simulink library "mdderslib_conversions"  (Simulink 7.8)
settings: Solver=ode45  StartTime=0.0  StopTime=10.0  RelTol=1e-3
settings Model: Creator=Tomas  LastModifiedBy=bures

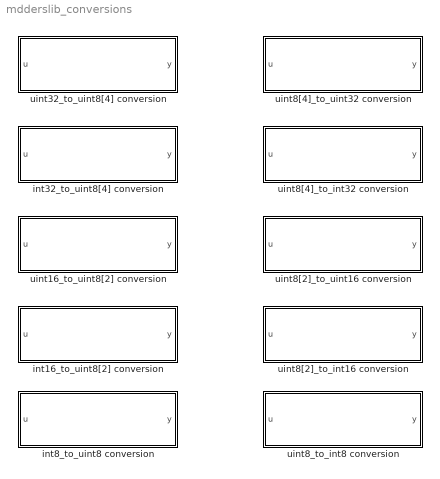
== system mdderslib_conversions ==
  int16_to_uint8[2] conversion : MATLAB Function  TreatAsAtomicUnit=on
  int32_to_uint8[4] conversion : MATLAB Function  TreatAsAtomicUnit=on
  int8_to_uint8 conversion : MATLAB Function  TreatAsAtomicUnit=on
  uint16_to_uint8[2] conversion : MATLAB Function  TreatAsAtomicUnit=on
  uint32_to_uint8[4] conversion : MATLAB Function  TreatAsAtomicUnit=on
  uint8[2]_to_int16 conversion : MATLAB Function  TreatAsAtomicUnit=on
  uint8[2]_to_uint16 conversion : MATLAB Function  TreatAsAtomicUnit=on
  uint8[4]_to_int32 conversion : MATLAB Function  TreatAsAtomicUnit=on
  uint8[4]_to_uint32 conversion : MATLAB Function  TreatAsAtomicUnit=on
  uint8_to_int8 conversion : MATLAB Function  TreatAsAtomicUnit=on

== matlab function uint32_to_uint8[4] conversion ==
  data: u input uint32 size=[1 1]; y output uint8 size=[1 4]
function y = uint32_to_uint8(u)
%#codegen

y = typecast(uint32(u), 'uint8');

== matlab function int32_to_uint8[4] conversion ==
  data: u input int32 size=[1 1]; y output uint8 size=[1 4]
function y = int32_to_uint8(u)
%#codegen

y = typecast(int32(u), 'uint8');

== matlab function int16_to_uint8[2] conversion ==
  data: u input int16 size=[1 1]; y output uint8 size=[1 2]
function y = int16_to_uint8(u)
%#codegen

y = typecast(int16(u), 'uint8');

== matlab function uint16_to_uint8[2] conversion ==
  data: u input uint16 size=[1 1]; y output uint8 size=[1 2]
function y = uint16_to_uint8(u)
%#codegen

y = typecast(uint16(u), 'uint8');

== matlab function uint8_to_int8 conversion ==
  data: u input uint8 size=[1 1]; y output int8 size=[1 1]
function y = uint8_to_int8(u)
%#codegen

y = typecast(uint8(u), 'int8');

== matlab function uint8[4]_to_int32 conversion ==
  data: u input uint8 size=[1 4]; y output int32 size=[1 1]
function y = uint8_to_int32(u)
%#codegen

y = typecast(uint8(u), 'int32');

== matlab function uint8[2]_to_uint16 conversion ==
  data: u input uint8 size=[1 2]; y output uint16 size=[1 1]
function y = uint8_to_uint16(u)
%#codegen

y = typecast(uint8(u), 'uint16');

== matlab function uint8[4]_to_uint32 conversion ==
  data: u input uint8 size=[1 4]; y output uint32 size=[1 1]
function y = uint8_to_uint32(u)
%#codegen

y = typecast(uint8(u), 'uint32');

== matlab function int8_to_uint8 conversion ==
  data: u input int8 size=[1 1]; y output uint8 size=[1 1]
function y = int8_to_uint8(u)
%#codegen

y = typecast(int8(u), 'uint8');

== matlab function uint8[2]_to_int16 conversion ==
  data: u input uint8 size=[1 2]; y output int16 size=[1 1]
function y = uint8_to_int16(u)
%#codegen

y = typecast(uint8(u), 'int16');
